simulink model "controller2_SR"  (R2020a)
settings: Solver=VariableStepAuto  StartTime=0.0  StopTime=30.0  RelTol=1e-3
values from neighbouring files (symbols this model uses):
  A = [0,       1 ... (first row only)    [capt_init_model.m]
  B = [0 ... (first row only)    [capt_init_model.m]
  C = [1, 0]    [capt_init_model.m]
  D = 0    [capt_init_model.m]
undefined symbols (not defined in the file or in its folder): b, den_d, DiscIntNeverNeededParam, k, num_d, omega_c, Ts
libraries: simulink x1, etargetslib x1, instrumentlib x1
settings Model: Creator=javot  LastModifiedBy=javot

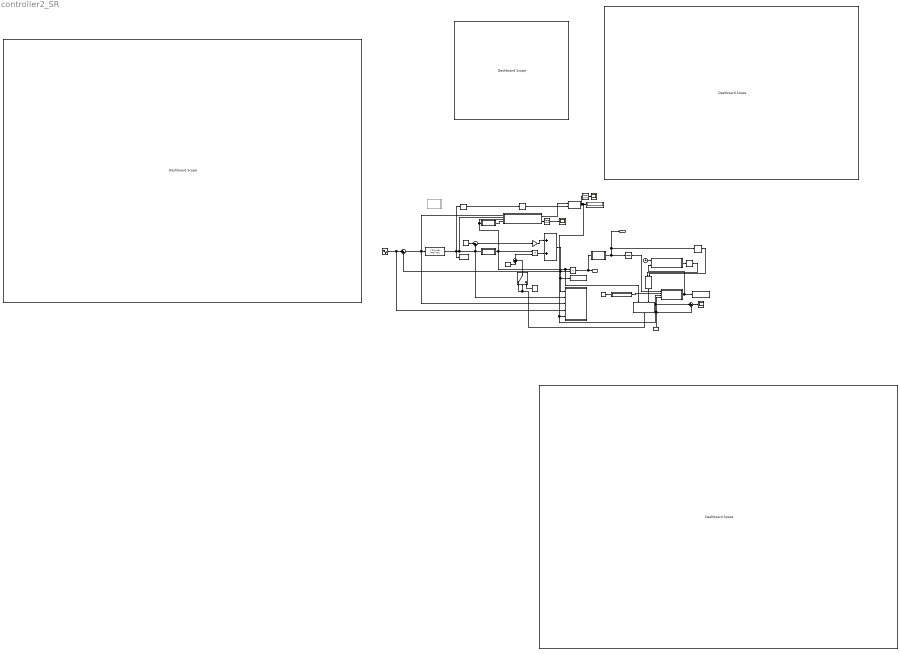
== system controller2_SR ==
  Add : Sum
  Cast To Double1 : DataTypeConversion  OutDataTypeStr=double
  Clock : Clock
  Constant2 : Constant  Value=0
  Dashboard Scope{,1..3} (4 alike) : DashboardScope
  Delay : Delay  DelayLength=1
  Delay1 : Delay  DelayLength=1
  Discrete-Time Integrator : DiscreteIntegrator  gainval=deltaT  SampleTime=-1  ICPrevOutput=DiscIntNeverNeededParam  ICPrevScaledInput=DiscIntNeverNeededParam
  Display : Display
  Energy_observer : MATLAB Function  TreatAsAtomicUnit=on
  Hit Crossing : HitCross
  Init_virtual_damping : Constant  Value=b
  MinMax Running Resettable : simulink/Math Operations/MinMax Running Resettable  Function=max  vinit=0.0
  Motor_state_space : StateSpace  A=A  B=B  C=C  D=D  InitialCondition=0  ContinuousStateAttributes="\"\""
  Product : Product
  Product2 : Product
  Rate Limiter : RateLimiter  SampleTimeMode=inherited
  Rate Limiter1 : RateLimiter  SampleTimeMode=inherited
  Scope13 : Scope
  Scope6 : Scope
  Subsystem : Subsystem
  Sum : Sum  Inputs=|++
  Sum1 : Sum  Inputs=|+-
  Sum2 : Sum  Inputs=|-+
  Sum4 : Sum  Inputs=|+-
  Switch1 : Switch  Criteria=u2 > Threshold  Threshold=0.001
  System_matrix : Constant  Value=A
  Time_window_est : MATLAB Function  TreatAsAtomicUnit=on
  Tw : ToWorkspace  VariableName=tw  SaveFormat=Timeseries  SampleTime=-1
  angle : ToWorkspace  VariableName=angle  SaveFormat=Timeseries  SampleTime=-1
  dominant_system_eigs : MATLAB Function  TreatAsAtomicUnit=on
  energy_trigger : MATLAB Function  TreatAsAtomicUnit=on
  impd_mismatch : Scope
  impedance_estimation : MATLAB Function  TreatAsAtomicUnit=on
  inital_excitation : Sin  SampleTime=Ts
  inject_cycle : MATLAB Function  TreatAsAtomicUnit=on
  kappas : Constant  Value=13.14
  number_crossings_zero : MATLAB Function  Commented=on  TreatAsAtomicUnit=on
  smooth_derivative : Subsystem
  smooth_derivative1 : Subsystem
  stiffness : Gain  Gain=k
  theta_ref : Constant  Value=0
  to_be_transm_outputs : Subsystem
  torque : ToWorkspace  VariableName=torque  SaveFormat=Timeseries  SampleTime=-1
  Running_energy : Outport
  Observed_energy : Outport  Port=2
  wires:
  Sum2/1 -> stiffness/1  "theta_error"
  Sum1/1 -> to_be_transm_outputs/3(state_in), Motor_state_space/1, impedance_estimation/1(tau_h)
  stiffness/1 -> Add/1
  Energy_observer/1(y) -> Delay/1, Observed_energy/1, Discrete-Time Integrator/1
  Product/1 -> Energy_observer/1(e_n), Running_energy/1
  Motor_state_space/1 -> impedance_estimation/2(theta), smooth_derivative/1(theta), to_be_transm_outputs/2(theta), Sum2/2, angle/1, Hit Crossing/1  "theta"
  Add/1 -> Product/2, Sum1/2, torque/1, to_be_transm_outputs/1(saturated_torque)
  Product2/1 -> Add/2
  theta_ref/1 -> Sum2/1
  Init_virtual_damping/1 -> Sum/1
  Sum/1 -> Product2/2  "total_damping"
  System_matrix/1 -> dominant_system_eigs/1(A)
  dominant_system_eigs/1(lambda_dom) -> Time_window_est/2(lambda_d)
  Time_window_est/1(time_win) -> Tw/1, inject_cycle/2(tw)  "Tw"
  Switch1/1 -> Sum/2
  Constant2/1 -> Switch1/3
  Discrete-Time Integrator/1 -> Time_window_est/1(E_err)
  Delay/1 -> energy_trigger/2(energy_in)
  energy_trigger/1(Einj) -> Subsystem/2(In2)
  inject_cycle/1(track_energy_cycle) -> Delay1/1
  Delay1/1 -> energy_trigger/1(trigger)
  Subsystem/1(Adaptive_damping) -> Switch1/1, Switch1/2  "extra_damping"
  Sum4/1 -> impd_mismatch/1
  kappas/1 -> Time_window_est/4(Zd), Sum4/2
  Clock/1 -> inject_cycle/1(time)
  inital_excitation/1 -> to_be_transm_outputs/4(init_excitation), Sum1/1
  smooth_derivative/1(theta_dot) -> Product2/1, Subsystem/1(omega), Product/1, impedance_estimation/3(omega), smooth_derivative1/1(theta)
  smooth_derivative1/1(theta_dot) -> impedance_estimation/4(alpha_acc)
  impedance_estimation/1(k_theta_est) -> MinMax Running Resettable/1
  Cast To Double1/1 -> MinMax Running Resettable/2  "reset_signal"
  MinMax Running Resettable/1 -> Rate Limiter/1, Sum4/1, Time_window_est/3(Z), to_be_transm_outputs/5(impedance), Display/1
  Hit Crossing/1 -> Cast To Double1/1
  Rate Limiter/1 -> Scope6/1
  impedance_estimation/2(b_theta_est) -> Rate Limiter1/1
  Rate Limiter1/1 -> Scope13/1

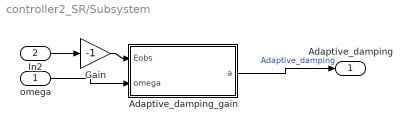
== system controller2_SR/Subsystem ==
  omega : Inport
  In2 : Inport  Port=2
  Adaptive_damping_gain : MATLAB Function  TreatAsAtomicUnit=on
  Gain : Gain  Gain=-1
  Adaptive_damping : Outport
  wires:
  In2/1 -> Gain/1
  Gain/1 -> Adaptive_damping_gain/1(Eobs)
  Adaptive_damping_gain/1(a) -> Adaptive_damping/1  "Adaptive_damping"
  omega/1 -> Adaptive_damping_gain/2(omega)

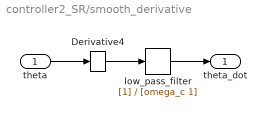
== system controller2_SR/smooth_derivative ==
  theta : Inport
  Derivative4 : Derivative
  low_pass_filter : TransferFcn  Denominator=[omega_c 1]
  theta_dot : Outport
  wires:
  Derivative4/1 -> low_pass_filter/1
  theta/1 -> Derivative4/1
  low_pass_filter/1 -> theta_dot/1

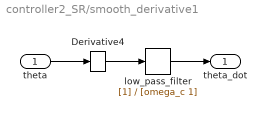
== system controller2_SR/smooth_derivative1 ==
  theta : Inport
  Derivative4 : Derivative
  low_pass_filter : TransferFcn  Denominator=[omega_c 1]
  theta_dot : Outport
  wires:
  Derivative4/1 -> low_pass_filter/1
  theta/1 -> Derivative4/1
  low_pass_filter/1 -> theta_dot/1

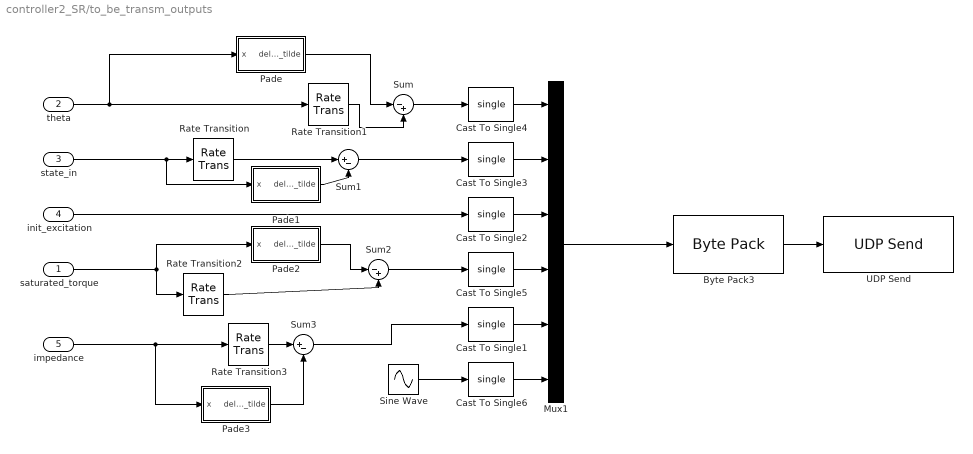
== system controller2_SR/to_be_transm_outputs ==
  saturated_torque : Inport
  theta : Inport  Port=2
  state_in : Inport  Port=3
  init_excitation : Inport  Port=4
  impedance : Inport  Port=5
  Byte Pack3 : etargetslib/Byte Pack  datatypes={'single'}  byteAlign=1
  Cast To Single{1..6} (6 alike) : DataTypeConversion  OutDataTypeStr=single
  Mux1 : Mux  Inputs=6
  Pade : Subsystem
  Pade1 : Subsystem
  Pade2 : Subsystem
  Pade3 : Subsystem
  Rate Transition{,1..3} (4 alike) : RateTransition
  Sine Wave : Sin  SampleTime=0.001
  Sum : Sum  Inputs=|-+
  Sum1 : Sum  Inputs=|+-
  Sum2 : Sum  Inputs=|-+
  Sum3 : Sum  Inputs=|+-
  UDP Send : instrumentlib/UDP Send  Host=134.105.60.99  Port=55001  LocalPort=-1  EnablePortSharing=off  ByteOrder=BigEndian  OutputDatagramPacketSize=512  EnableBlockingMode=on  LocalAddress=0.0.0.0
  wires:
  Byte Pack3/1 -> UDP Send/1
  Mux1/1 -> Byte Pack3/1
  Sine Wave/1 -> Cast To Single6/1
  init_excitation/1 -> Cast To Single2/1
  theta/1 -> Pade/1(x), Rate Transition1/1
  saturated_torque/1 -> Pade2/1(x), Rate Transition2/1
  impedance/1 -> Pade3/1(x), Rate Transition3/1
  Cast To Single4/1 -> Mux1/1
  Cast To Single3/1 -> Mux1/2
  Cast To Single5/1 -> Mux1/4
  Cast To Single2/1 -> Mux1/3
  Cast To Single1/1 -> Mux1/5
  Cast To Single6/1 -> Mux1/6
  Rate Transition1/1 -> Sum/2
  Sum/1 -> Cast To Single4/1
  Rate Transition/1 -> Sum1/1
  Sum1/1 -> Cast To Single3/1
  Rate Transition2/1 -> Sum2/2
  Sum2/1 -> Cast To Single5/1
  Rate Transition3/1 -> Sum3/1
  Sum3/1 -> Cast To Single1/1
  state_in/1 -> Pade1/1(x), Rate Transition/1
  Pade2/1(delay_tilde) -> Sum2/1
  Pade/1(delay_tilde) -> Sum/1
  Pade1/1(delay_tilde) -> Sum1/2
  Pade3/1(delay_tilde) -> Sum3/2

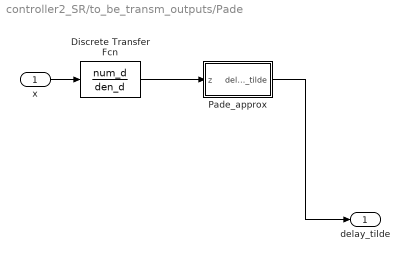
== system controller2_SR/to_be_transm_outputs/Pade ==
  x : Inport
  Discrete Transfer Fcn : DiscreteTransferFcn  Numerator=num_d  Denominator=den_d
  Pade_approx : MATLAB Function  TreatAsAtomicUnit=on
  delay_tilde : Outport
  wires:
  Discrete Transfer Fcn/1 -> Pade_approx/1(z)
  Pade_approx/1(delay_tilde) -> delay_tilde/1
  x/1 -> Discrete Transfer Fcn/1

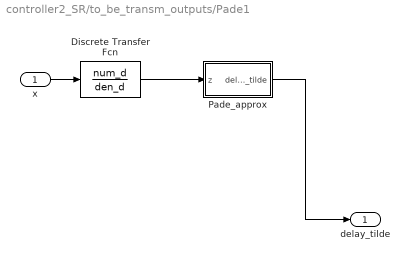
== system controller2_SR/to_be_transm_outputs/Pade1 ==
  x : Inport
  Discrete Transfer Fcn : DiscreteTransferFcn  Numerator=num_d  Denominator=den_d
  Pade_approx : MATLAB Function  TreatAsAtomicUnit=on
  delay_tilde : Outport
  wires:
  Discrete Transfer Fcn/1 -> Pade_approx/1(z)
  Pade_approx/1(delay_tilde) -> delay_tilde/1
  x/1 -> Discrete Transfer Fcn/1

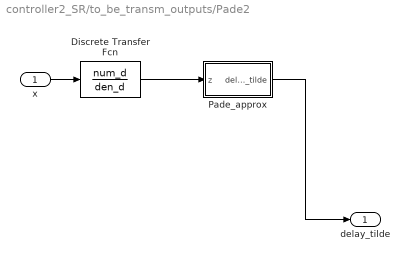
== system controller2_SR/to_be_transm_outputs/Pade2 ==
  x : Inport
  Discrete Transfer Fcn : DiscreteTransferFcn  Numerator=num_d  Denominator=den_d
  Pade_approx : MATLAB Function  TreatAsAtomicUnit=on
  delay_tilde : Outport
  wires:
  Discrete Transfer Fcn/1 -> Pade_approx/1(z)
  Pade_approx/1(delay_tilde) -> delay_tilde/1
  x/1 -> Discrete Transfer Fcn/1

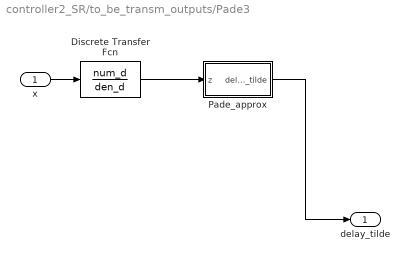
== system controller2_SR/to_be_transm_outputs/Pade3 ==
  x : Inport
  Discrete Transfer Fcn : DiscreteTransferFcn  Numerator=num_d  Denominator=den_d
  Pade_approx : MATLAB Function  TreatAsAtomicUnit=on
  delay_tilde : Outport
  wires:
  Discrete Transfer Fcn/1 -> Pade_approx/1(z)
  Pade_approx/1(delay_tilde) -> delay_tilde/1
  x/1 -> Discrete Transfer Fcn/1

== matlab function controller2_SR/number_crossings_zero ==
  settings: updateMethod=DISCRETE
  data: angle input; crossings output
function crossings = fcn(angle)

persistent prev_angle crossings_count

if isempty(prev_angle)
    prev_angle = angle;
    crossings_count = 0;
end

% Detect sign change (zero crossing)
if (angle > 0 && prev_angle < 0) || (angle < 0 && prev_angle > 0)
    crossings_count = crossings_count + 1;
end

% Update previous value
prev_angle = angle;

% Output
crossings = crossings_count;

end

== matlab function controller2_SR/to_be_transm_outputs/Pade1/Pade_approx ==
  data: delay_tilde output; z input
function delay_tilde= fcn(z)
persistent z_prev; 
persistent delay_prev;

if isempty(z_prev)
    z_prev = 0;
    delay_prev = 0;
end
delay_tilde = z/3 + z_prev + (1/3)*delay_prev;
z_prev = z;
delay_prev = delay_tilde;

end

== matlab function controller2_SR/to_be_transm_outputs/Pade/Pade_approx ==
  data: delay_tilde output; z input
function delay_tilde= fcn(z)
persistent z_prev; 
persistent delay_prev;

if isempty(z_prev)
    z_prev = 0;
    delay_prev = 0;
end
delay_tilde = z/3 + z_prev + (1/3)*delay_prev;
z_prev = z;
delay_prev = delay_tilde;

end

== matlab function controller2_SR/to_be_transm_outputs/Pade2/Pade_approx ==
  data: delay_tilde output; z input
function delay_tilde= fcn(z)
persistent z_prev; 
persistent delay_prev;

if isempty(z_prev)
    z_prev = 0;
    delay_prev = 0;
end
delay_tilde = z/3 + z_prev + (1/3)*delay_prev;
z_prev = z;
delay_prev = delay_tilde;

end

== matlab function controller2_SR/to_be_transm_outputs/Pade3/Pade_approx ==
  data: delay_tilde output; z input
function delay_tilde= fcn(z)
persistent z_prev; 
persistent delay_prev;

if isempty(z_prev)
    z_prev = 0;
    delay_prev = 0;
end
delay_tilde = z/3 + z_prev + (1/3)*delay_prev;
z_prev = z;
delay_prev = delay_tilde;

end

== matlab function controller2_SR/Energy_observer ==
  settings: updateMethod=DISCRETE
  data: e_n input; y output
function y = fcn(e_n)

persistent e_prev

if isempty(e_prev)
    e_prev = 0.01;      % initial condition
end

y = e_n - e_prev;

e_prev = y;

== matlab function controller2_SR/inject_cycle ==
  settings: updateMethod=DISCRETE
  data: time input; track_energy_cycle output; tw input
function track_energy_cycle  = fcn(time, tw)

%Induction on time window 
persistent start_time 

if isempty(start_time)
    start_time = 0.0;
end 
if time-start_time>tw 
    track_energy_cycle = true;
    start_time = time;
else
    track_energy_cycle = false;
end 

end

== matlab function controller2_SR/Subsystem/Adaptive_damping_gain ==
  settings: updateMethod=DISCRETE
  data: Eobs input; a output; omega input
function a = fcn(Eobs, omega)

persistent a_prev

% Parameters
deltaT = 0.001;
omega_min = 1e-3;     % Prevent division by zero
a_min = 0.001;
a_max = 100;          

% Initialization
if isempty(a_prev)
    a_prev = 1e-4;
end

% Safe angular velocity
omega_safe = max(abs(omega), omega_min);

% Adaptation law
if Eobs < 0
    a = a_prev + Eobs/(deltaT*omega_safe^2);
else
    % Keep previous value instead of resetting
    a = a_prev;
end

% Saturation
a = min(max(a, a_min), a_max);

% Store for next iteration
a_prev = a;

end

== matlab function controller2_SR/Time_window_est ==
  settings: updateMethod=DISCRETE
  data: E_err input; time_win output; lambda_d input; Z input; Zd input
function time_win = Time_window_est(E_err, lambda_d, Z, Zd)
%#codegen
% TIME_WINDOW_EST Adaptive observation window estimator using 5-sample time-window
% local minimum detection based on Dinc et al. (IEEE TOH 2024).
%
% Inputs:
%   E_err    : Accumulated energy error/net energy [J]
%   lambda_d : Desired system eigenvalue / dynamic pole
%   Z        : Current impedance estimate
%   Zd       : Target/desired impedance
%
% Output:
%   time_win : Adaptive time window duration [s]

persistent E_window      % 5-sample window: [E(t-2), E(t-1), E(t), E(t+1), E(t+2)]
persistent t_prev        % Previous smoothed window output

%% Limits & Reference Gains
Tmin = 0.01;            % Minimum window time [s]
Tmax = 0.50;            % Maximum window time [s]

tau_min = Tmin;
tau_max = Tmax;

Eref = 1e-3;
k_energy = 0.8;
k_impedance = 0.8;
alpha_time = 0.25;      % Smoothing filter factor

%% Initialization
if isempty(E_window)
    E_window = zeros(5, 1);
    t_prev   = 0.1;
end

%% 1. Slide 5-Sample Time-Window (Fig. 4)
% Shift energy history left: t-2 <- t-1 <- t <- t+1 <- t+2
E_window(1) = E_window(2);
E_window(2) = E_window(3);
E_window(3) = E_window(4);
E_window(4) = E_window(5);
E_window(5) = E_err;

%% 2. Time-Window Local Minimum Detection (Eq. 10)
% Condition: E(t-2) > E(t-1) > E(t) < E(t+1) < E(t+2)
% Validates true energy cycle transition without noise-induced false triggers
is_cycle_min = (E_window(1) > E_window(2)) && ...
               (E_window(2) > E_window(3)) && ...
               (E_window(3) < E_window(4)) && ...
               (E_window(4) < E_window(5));

%% 3. System Time Constant Calculation
lambda_real = real(lambda_d);

if lambda_real < -1e-6
    tau_c = -1/lambda_real;
else
    tau_c = tau_max;
end

tau_c = min(max(tau_c, tau_min), tau_max);

%% 4. Normalized Error & Impedance Mismatch
energy_error = abs(E_err) / max(Eref, 1e-12);
impedance_error = norm(Z - Zd) / (norm(Zd) + 1e-12);

% Saturation bounds
energy_error = min(energy_error, 5.0);
impedance_error = min(impedance_error, 5.0);

%% 5. Adaptive Window Scaling (Integrating Paper's Cycle Detection)
% Basic error factor based on energy and impedance mismatch
error_factor = 1.0 / (1.0 + k_energy * energy_error + k_impedance * impedance_error);

% If time-window validates an energy cycle completion (local minimum),
% we confirm dynamic stability and scale toward the nominal target window.
if is_cycle_min
    cycle_factor = 1.0; 
else
    % During transient/noisy phases without cycle minimum, reduce window size
    cycle_factor = 0.5; 
end

% Combine candidate time window
time_candidate = tau_c * error_factor * cycle_factor;
time_candidate = min(max(time_candidate, Tmin), Tmax);

%% 6. Smooth Output Transition
time_win = (1.0 - alpha_time) * t_prev + alpha_time * time_candidate;
time_win = min(max(time_win, Tmin), Tmax);

t_prev = time_win;

end

== matlab function controller2_SR/dominant_system_eigs ==
  data: A input; lambda_dom output
function lambda_dom = fcn(A)

%Fetch eigs of system matrix and find the dominant one 
lambdas = eig(A);
[~, idx]= max(real(lambdas));
lambda_dom = lambdas(idx);

== matlab function controller2_SR/impedance_estimation ==
  settings: updateMethod=DISCRETE
  data: tau_h input; theta input; omega input; alpha_acc input; k_theta_est output; b_theta_est output
function [k_theta_est, b_theta_est] = fcn(tau_h, theta, omega, alpha_acc)
%#codegen

    % Persistent variables for RLS estimation memory
    persistent Theta P initialized
    
    % Configuration Parameters
    J = 0.0103;                % Device rotational inertia (kg*m^2)
    
    % Initialization on the first step
    if isempty(initialized)
        Theta = [0.0; 0.0];    % Initial parameter vector [k; b] starting at zero
        P = 100 * eye(2);      % Initial covariance matrix
        initialized = true;
    end
    
    % Default outputs to current estimates
    k_theta_est = Theta(1);
    b_theta_est = Theta(2);
    
    % Active motion and excitation check (prevents division by zero / noise drift)
    if abs(omega) > 0.005 || abs(theta) > 0.005
        
        % Regressor vector containing the independent variables [theta; omega]
        phi = [theta; omega];
        
        % Measured net torque available for spring and damper absorption
        y = tau_h - J * alpha_acc;
        
        % RLS Algorithm with Forgetting Factor (lambda)
        lambda = 0.98;         % Memory weighting (lower = faster tracking, higher = smoother)
        
        denominator = lambda + phi' * P * phi;
        
        if denominator > 1e-5
            % Compute Kalman-like gain vector
            K_gain = (P * phi) / denominator;
            
            % Prediction error based on current parameter guesses
            prediction_error = y - phi' * Theta;
            
            % Update parameter estimates [k; b]
            Theta = Theta + K_gain * prediction_error;
            
            % Update and bound covariance matrix P to prevent windup/explosion
            P_new = (P - K_gain * phi' * P) / lambda;
            if trace(P_new) < 1e5 && all(isfinite(P_new(:)))
                P = P_new;
            else
                P = 100 * eye(2); % Reset covariance safely if it tries to grow
            end
        end
        
    else
        % When inactive/stopped, gently leak/decay parameters back to zero
        decay = 0.02;
        Theta = Theta * (1 - decay);
    end
    
    % Strict physical bounding to guarantee meaningful and safe values
    k_theta_est = min(max(0, Theta(1)), 50000); % Bounded between 0 and 50,000 Nm/rad
    b_theta_est = min(max(0, Theta(2)), 200);   % Bounded between 0 and 200 Nms/rad
    
    % Final NaN/Inf safety net
    if ~isfinite(k_theta_est), k_theta_est = 0; end
    if ~isfinite(b_theta_est), b_theta_est = 0; end
    
    % Update persistent state vector
    Theta(1) = k_theta_est;
    Theta(2) = b_theta_est;
     % Low-pass filtering coefficient (closer to 1 = smoother, closer to 0 = faster)
    alpha_smooth = 0.05; 
     % Persistent variables for internal low-pass smoothing
    persistent k_filtered b_filtered
    if isempty(k_filtered)
        k_filtered = 0;
        b_filtered = 0;
    end
    
    k_filtered = (1 - alpha_smooth) * k_filtered + alpha_smooth * k_theta_est;
    b_filtered = (1 - alpha_smooth) * b_filtered + alpha_smooth * b_theta_est;
    
    % Final output assignment
    k_theta_est = k_filtered;
    b_theta_est = b_filtered;
end

== matlab function controller2_SR/energy_trigger ==
  data: trigger input; Einj output; energy_in input
function Einj = fcn(trigger, energy_in)

if trigger == true
    Einj = energy_in;
else 
    Einj = 0;
end

end
